simulink model "Model_6DoF_Complete"  (R2024a)
settings: Solver=VariableStepAuto  StartTime=0.0  StopTime=6  RelTol=1e-5
model workspace: external: MATLAB File C:\Users\C27Derek.Weissinger\OneDrive - USAFA (AFAcademy.AF.edu)\Documents\Classes\Summer 26\Astro 499\Derek-Weissinger-GNC-Methods-2026\MATLAB + Simulink\vehicle_params.m (data not in the file)
undefined symbols (not defined in the file): I, Kd, Ki, Kp, Lg, m, psii, thetai, Ts
libraries: simulink_extras x10, eeGeneralControl x2, sharedtransform x2, shared6dof x1, sharedutil x1
settings Model: Creator=C28Derek.Weissinger  LastModifiedBy=C28Derek.Weissinger

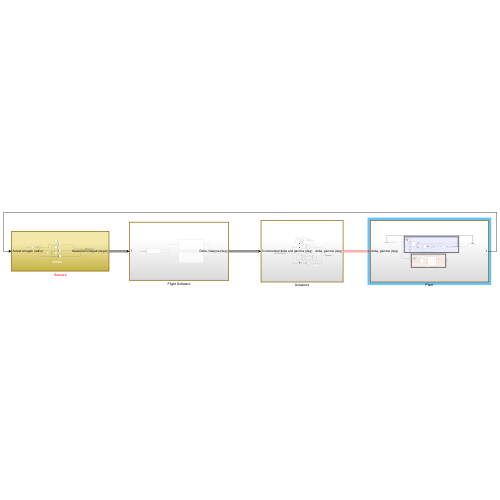
[thumbnail: Simulink's stored preview of the top-level diagram]
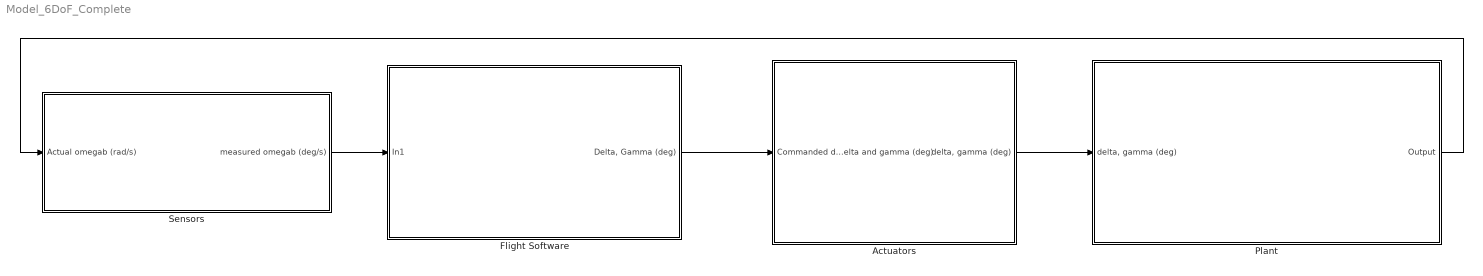
== system Model_6DoF_Complete ==
  Actuators : Subsystem
  Flight Software : Subsystem
  Plant : Subsystem
  Sensors : Subsystem
  wires:
  Plant/1(Output) -> Sensors/1(Actual omegab (rad/s))
  Sensors/1(measured omegab (deg/s)) -> Flight Software/1(In1)
  Flight Software/1("Delta, Gamma (deg)") -> Actuators/1(Commanded delta and gamma (deg))
  Actuators/1("delta, gamma (deg)") -> Plant/1("delta, gamma (deg)")

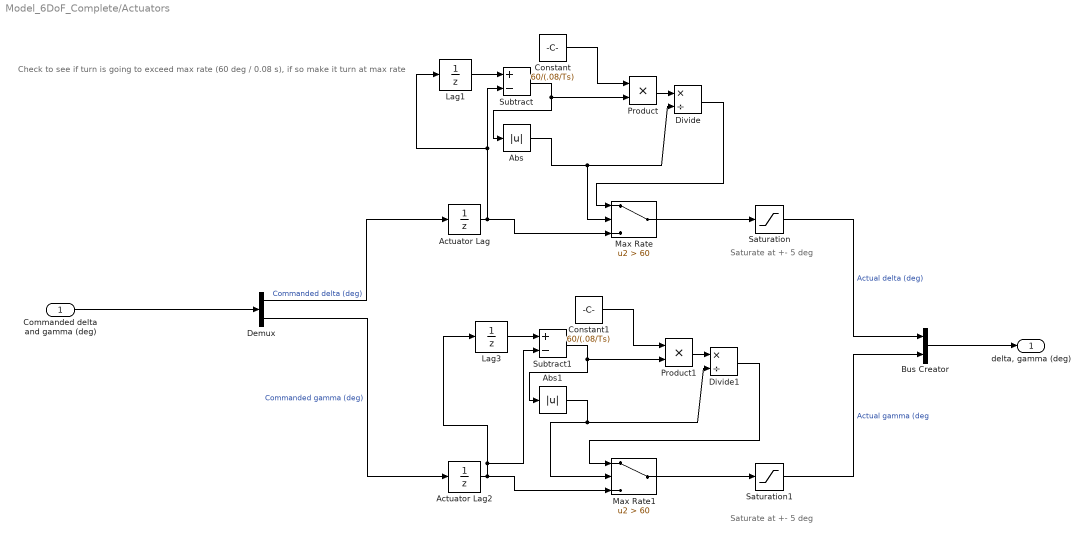
== system Model_6DoF_Complete/Actuators ==
  note: Saturate at +- 5 deg
  note: Check to see if turn is going to exceed max rate (60 deg / 0.08 s), if so make it turn at max rate
  note: Saturate at +- 5 deg
  Commanded delta and gamma (deg) : Inport
  Abs : Abs  SaturateOnIntegerOverflow=off
  Abs1 : Abs  SaturateOnIntegerOverflow=off
  Actuator Lag : UnitDelay  SampleTime=Ts  HasFrameUpgradeWarning=on
  Actuator Lag2 : UnitDelay  SampleTime=Ts  HasFrameUpgradeWarning=on
  Bus Creator : BusCreator  Inputs=2
  Constant : Constant  Value=60/(.08/Ts)
  Constant1 : Constant  Value=60/(.08/Ts)
  Demux : Demux  Outputs=2
  Divide : Product  Inputs=*/
  Divide1 : Product  Inputs=*/
  Lag1 : UnitDelay  SampleTime=0.08  HasFrameUpgradeWarning=on
  Lag3 : UnitDelay  SampleTime=0.08  HasFrameUpgradeWarning=on
  Max Rate : Switch  Criteria=u2 > Threshold  Threshold=60  SaturateOnIntegerOverflow=off  InputSameDT=off
  Max Rate1 : Switch  Criteria=u2 > Threshold  Threshold=60  SaturateOnIntegerOverflow=off  InputSameDT=off
  Product : Product
  Product1 : Product
  Saturation : Saturate  UpperLimit=5  LowerLimit=-5
  Saturation1 : Saturate  UpperLimit=5  LowerLimit=-5
  Subtract : Sum  Inputs=+-
  Subtract1 : Sum  Inputs=+-
  "delta, gamma (deg)" : Outport
  wires:
  Actuator Lag/1 -> Max Rate/3, Subtract/2, Lag1/1
  Lag1/1 -> Subtract/1
  Subtract/1 -> Abs/1, Product/2
  Abs/1 -> Max Rate/2, Divide/2
  Constant/1 -> Product/1
  Product/1 -> Divide/1
  Max Rate/1 -> Saturation/1
  Saturation1/1 -> Bus Creator/2  "Actual gamma (deg"
  Max Rate1/1 -> Saturation1/1
  Subtract1/1 -> Abs1/1, Product1/2
  Abs1/1 -> Max Rate1/2, Divide1/2
  Actuator Lag2/1 -> Max Rate1/3, Subtract1/2, Lag3/1
  Demux/2 -> Actuator Lag2/1  "Commanded gamma (deg)"
  Product1/1 -> Divide1/1
  Constant1/1 -> Product1/1
  Lag3/1 -> Subtract1/1
  Demux/1 -> Actuator Lag/1  "Commanded delta (deg)"
  Commanded delta and gamma (deg)/1 -> Demux/1
  Bus Creator/1 -> "delta, gamma (deg)"/1
  Saturation/1 -> Bus Creator/1  "Actual delta (deg)"
  Divide1/1 -> Max Rate1/1
  Divide/1 -> Max Rate/1

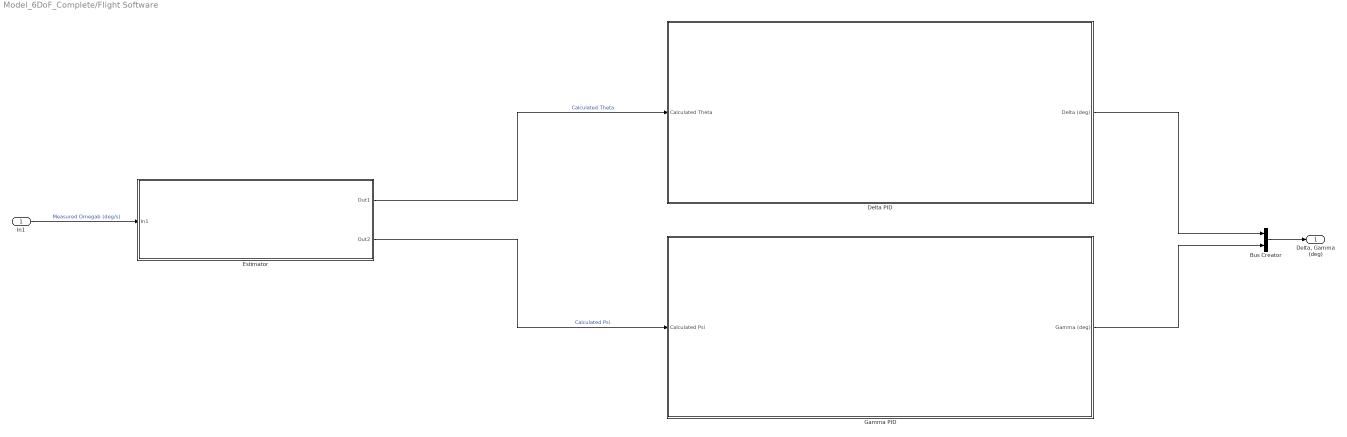
== system Model_6DoF_Complete/Flight Software ==
  In1 : Inport
  Bus Creator : BusCreator  Inputs=2
  Delta PID : Subsystem
  Estimator : Subsystem
  Gamma PID : Subsystem
  "Delta, Gamma (deg)" : Outport
  wires:
  In1/1 -> Estimator/1(In1)  "Measured Omegab (deg/s)"
  Bus Creator/1 -> "Delta, Gamma (deg)"/1
  Delta PID/1(Delta (deg)) -> Bus Creator/1
  Gamma PID/1(Gamma (deg)) -> Bus Creator/2
  Estimator/1(Out1) -> Delta PID/1(Calculated Theta)  "Calculated Theta"
  Estimator/2(Out2) -> Gamma PID/1(Calculated Psi)  "Calculated Psi"

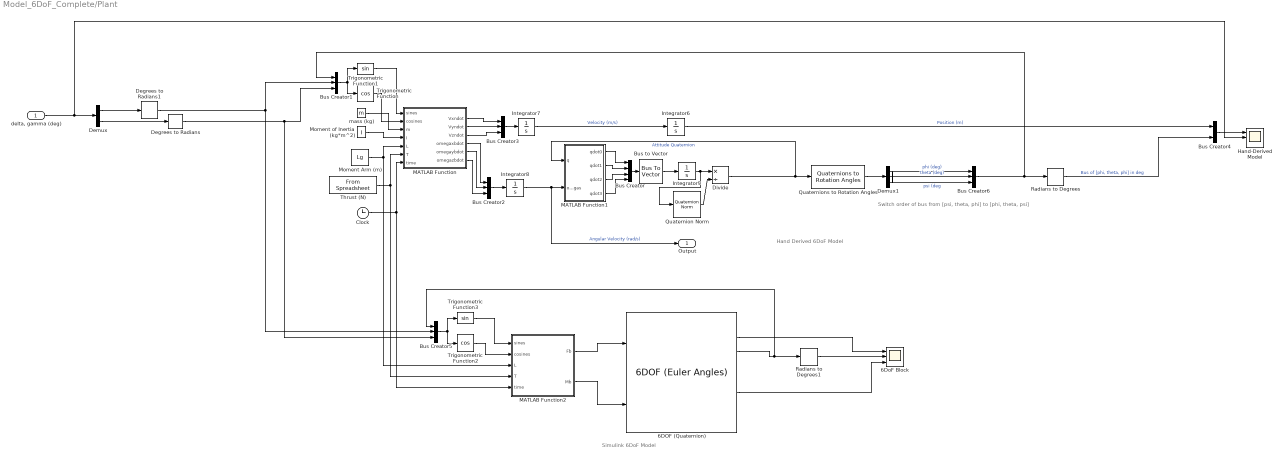
== system Model_6DoF_Complete/Plant ==
  note: Hand Derived 6DoF Model
  note: Simulink 6DoF Model
  note: Switch order of bus from [psi, theta, phi] to [phi, theta, psi]
  "delta, gamma (deg)" : Inport
  6DOF (Quaternion) : shared6dof/6DOF (Euler Angles)  units=Metric (MKS)  mtype=Fixed  rep=Quaternion  xme_0=[0 0 0]  Vm_0=[0 0 0]  eul_0=[0 deg2rad(thetai) deg2rad(psii)]  pm_0=[0 0 0]  mass_0=m  mass_e=0.5  mass_f=2.0  inertia=eye(3) * I  inertia_e=eye(3)  inertia_f=2*eye(3)  k_quat=1.0  vre_flag=on  abi_flag=off  aMode=0  xme_statename=''  Vm_statename=''  eul_statename=''  quat_statename=''  pm_statename=''  mass_statename=''
      settings: LibrarySourceBlock=aerolib6dof2/6DOF (Quaternion)
  6DoF Block : Scope  NumInputPorts=3
  Bus Creator : BusCreator  Inputs=4
  Bus Creator{1..3,5..6} (5 alike) : BusCreator  Inputs=3
  Bus Creator4 : BusCreator  Inputs=2
  Bus to Vector : BusToVector
  Clock : Clock
  Degrees to Radians : simulink_extras/Transformations/Degrees to Radians
  Degrees to Radians1 : simulink_extras/Transformations/Degrees to Radians
  Demux : Demux  Outputs=2
  Demux1 : Demux  Outputs=3
  Divide : Product  Inputs=*/
  Hand-Derived Model : Scope  NumInputPorts=3
  Integrator6 : Integrator
  Integrator7 : Integrator  InitialCondition=[0, 0, 0]
  Integrator8 : Integrator  InitialCondition=[0, 0, 0]
  Integrator9 : Integrator  InitialCondition=eul2quat([deg2rad(psii),deg2rad(thetai),deg2rad(0)])
  MATLAB Function : MATLAB Function  TreatAsAtomicUnit=on
  MATLAB Function1 : MATLAB Function  TreatAsAtomicUnit=on
  MATLAB Function2 : MATLAB Function  TreatAsAtomicUnit=on
  Moment Arm (m) : Constant  Value=Lg
  Moment of Inertia (kg*m^2) : Constant  Value=I
  Quaternion Norm : sharedutil/Quaternion Norm  aMode=aMode
      settings: LibrarySourceBlock=|
      | aerolibutil/Quaternion
      | Norm
  Quaternions to Rotation Angles : sharedtransform/Quaternions to Rotation Angles  rotationOrder=ZYX  aMode=aMode
  Radians to Degrees : simulink_extras/Transformations/Radians to Degrees
  Radians to Degrees1 : simulink_extras/Transformations/Radians to Degrees
  Thrust (N) : FromSpreadsheet  FileName=Estes_F15.csv  SheetName=Estes_F15  ExtrapolationAfterLastDataPoint=Ground value
  Trigonometric Function : Trigonometry  Operator=cos
  Trigonometric Function1 : Trigonometry
  Trigonometric Function2 : Trigonometry  Operator=cos
  Trigonometric Function3 : Trigonometry
  mass (kg) : Constant  Value=m
  Output : Outport
  wires:
  "delta, gamma (deg)"/1 -> Hand-Derived Model/2, Demux/1
  Moment Arm (m)/1 -> MATLAB Function2/3(L), MATLAB Function/5(L)
  Moment of Inertia (kg*m^2)/1 -> MATLAB Function/4(I)
  Degrees to Radians/1 -> Bus Creator5/3, Bus Creator1/3
  Bus Creator1/1 -> Trigonometric Function/1, Trigonometric Function1/1
  Trigonometric Function1/1 -> MATLAB Function/1(sines)
  Trigonometric Function/1 -> MATLAB Function/2(cosines)
  Thrust (N)/1 -> MATLAB Function2/4(T), MATLAB Function/6(T)
  mass (kg)/1 -> MATLAB Function/3(m)
  MATLAB Function/1(Vxndot) -> Bus Creator3/1
  Integrator7/1 -> Integrator6/1  "Velocity (m/s)"
  Integrator6/1 -> Bus Creator4/1  "Position (m)"
  Integrator8/1 -> Output/1, MATLAB Function1/2(omegas)  "Angular Velocity (rad/s)"
  MATLAB Function1/1(qdot0) -> Bus Creator/1
  Bus Creator4/1 -> Hand-Derived Model/1
  Clock/1 -> MATLAB Function2/5(time), MATLAB Function/7(time)
  Degrees to Radians1/1 -> Bus Creator1/2, Bus Creator5/2
  MATLAB Function1/2(qdot1) -> Bus Creator/2
  MATLAB Function1/3(qdot2) -> Bus Creator/3
  MATLAB Function1/4(qdot3) -> Bus Creator/4
  Bus Creator/1 -> Bus to Vector/1
  Bus to Vector/1 -> Integrator9/1
  Bus Creator2/1 -> Integrator8/1
  MATLAB Function/4(omegaxbdot) -> Bus Creator2/1
  MATLAB Function/5(omegaybdot) -> Bus Creator2/2
  MATLAB Function/6(omegazbdot) -> Bus Creator2/3
  Bus Creator3/1 -> Integrator7/1
  MATLAB Function/2(Vyndot) -> Bus Creator3/2
  MATLAB Function/3(Vzndot) -> Bus Creator3/3
  Integrator9/1 -> Quaternion Norm/1, Divide/1
  Divide/1 -> MATLAB Function1/1(q), Quaternions to Rotation Angles/1  "Attitude Quaternion"
  Quaternion Norm/1 -> Divide/2
  Demux/2 -> Degrees to Radians/1
  Demux/1 -> Degrees to Radians1/1
  MATLAB Function2/1(Fb) -> 6DOF (Quaternion)/1
  MATLAB Function2/2(Mb) -> 6DOF (Quaternion)/2
  6DOF (Quaternion)/3 -> Bus Creator5/1, Radians to Degrees1/1
  Radians to Degrees1/1 -> 6DoF Block/2
  6DOF (Quaternion)/2 -> 6DoF Block/1
  6DOF (Quaternion)/6 -> 6DoF Block/3
  Bus Creator5/1 -> Trigonometric Function2/1, Trigonometric Function3/1
  Trigonometric Function3/1 -> MATLAB Function2/1(sines)
  Trigonometric Function2/1 -> MATLAB Function2/2(cosines)
  Radians to Degrees/1 -> Bus Creator4/2  "Bus of [phi, theta, phi] in deg"
  Demux1/2 -> Bus Creator6/2  "theta (deg)"
  Demux1/3 -> Bus Creator6/1  "phi (deg)"
  Demux1/1 -> Bus Creator6/3  "psi (deg"
  Quaternions to Rotation Angles/1 -> Demux1/1
  Bus Creator6/1 -> Bus Creator1/1, Radians to Degrees/1

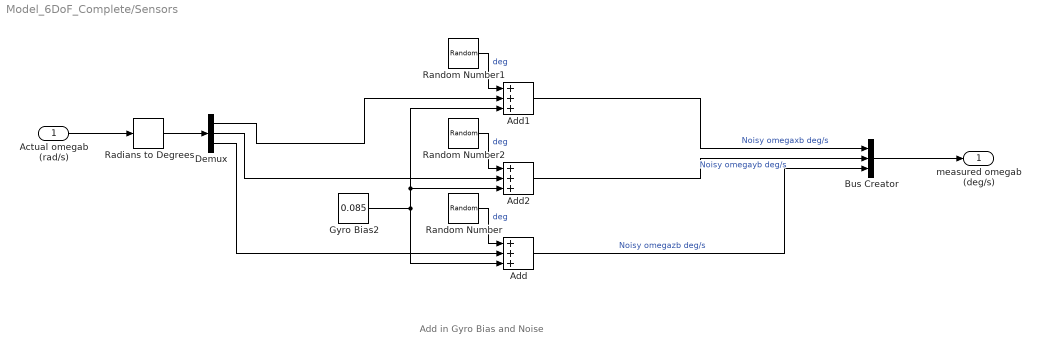
== system Model_6DoF_Complete/Sensors ==
  note: Add in Gyro Bias and Noise
  Actual omegab (rad/s) : Inport
  Add : Sum  Inputs=+++
  Add1 : Sum  Inputs=+++
  Add2 : Sum  Inputs=+++
  Bus Creator : BusCreator  Inputs=3
  Demux : Demux  Outputs=3
  Gyro Bias2 : Constant  Value=0.085
  Radians to Degrees : simulink_extras/Transformations/Radians to Degrees
  Random Number : RandomNumber  Seed=3  SampleTime=0.01
  Random Number1 : RandomNumber  Seed=1  SampleTime=0.01
  Random Number2 : RandomNumber  Seed=2  SampleTime=0.01
  measured omegab (deg/s) : Outport
  wires:
  Actual omegab (rad/s)/1 -> Radians to Degrees/1
  Random Number/1 -> Add/1  "deg"
  Add/1 -> Bus Creator/3  "Noisy omegazb deg/s"
  Bus Creator/1 -> measured omegab (deg/s)/1
  Add1/1 -> Bus Creator/1  "Noisy omegaxb deg/s"
  Random Number1/1 -> Add1/1  "deg"
  Gyro Bias2/1 -> Add1/3, Add2/3, Add/3
  Add2/1 -> Bus Creator/2  "Noisy omegayb deg/s"
  Random Number2/1 -> Add2/1  "deg"
  Demux/1 -> Add1/2
  Demux/2 -> Add2/2
  Demux/3 -> Add/2
  Radians to Degrees/1 -> Demux/1

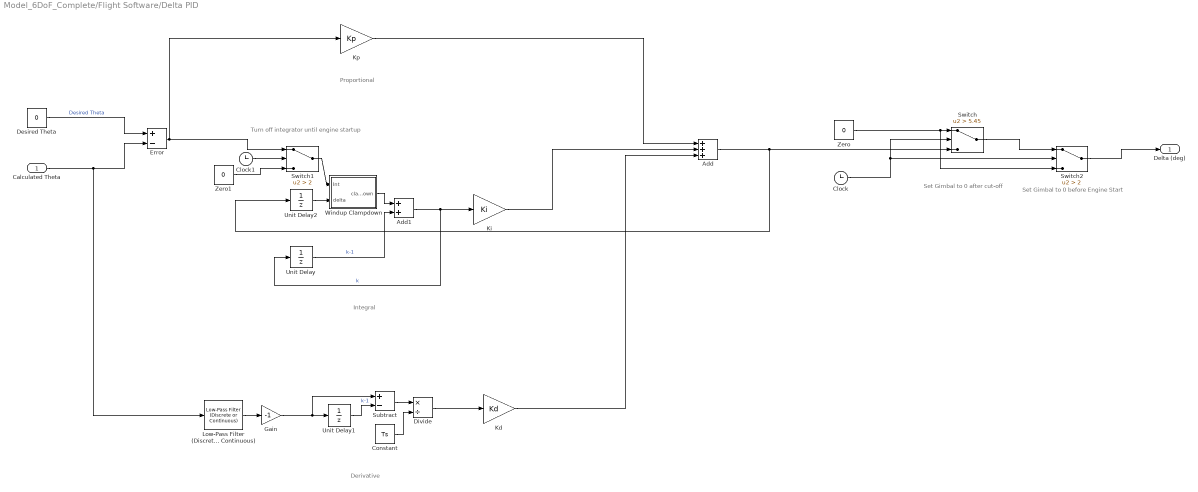
== system Model_6DoF_Complete/Flight Software/Delta PID ==
  note: Turn off integrator until engine startup
  note: Integral
  note: Proportional
  note: Derivative
  note: Set Gimbal to 0 before Engine Start
  note: Set Gimbal to 0 after cut-off
  Calculated Theta : Inport
  Add : Sum  Inputs=+++
  Add1 : Sum
  Clock : Clock
  Clock1 : Clock
  Constant : Constant  Value=Ts
  Desired Theta : Constant  Value=0
  Divide : Product  Inputs=*/
  Error : Sum  Inputs=+-
  Gain : Gain  Gain=-1
  Kd : Gain  Gain=Kd
  Ki : Gain  Gain=Ki
  Kp : Gain  Gain=Kp
  Low-Pass Filter (Discrete or Continuous) : eeGeneralControl/Low-Pass Filter (Discrete or Continuous)  K=1  T=2*Ts  B=inf  A=-inf  init_option=Inherited from block input  x0=0  Ts=-1
  Subtract : Sum  Inputs=+-
  Switch : Switch  Criteria=u2 > Threshold  Threshold=5.45  SaturateOnIntegerOverflow=off  InputSameDT=off
  Switch1 : Switch  Criteria=u2 > Threshold  Threshold=2  SaturateOnIntegerOverflow=off  InputSameDT=off
  Switch2 : Switch  Criteria=u2 > Threshold  Threshold=2  SaturateOnIntegerOverflow=off  InputSameDT=off
  Unit Delay : UnitDelay  SampleTime=Ts  HasFrameUpgradeWarning=on
  Unit Delay1 : UnitDelay  SampleTime=Ts  HasFrameUpgradeWarning=on
  Unit Delay2 : UnitDelay  SampleTime=Ts  HasFrameUpgradeWarning=on
  Windup Clampdown : MATLAB Function  TreatAsAtomicUnit=on
  Zero : Constant  Value=0  OutDataTypeStr=Inherit: Inherit via back propagation
  Zero1 : Constant  Value=0  OutDataTypeStr=Inherit: Inherit via back propagation
  Delta (deg) : Outport
  wires:
  Desired Theta/1 -> Error/1  "Desired Theta"
  Subtract/1 -> Divide/1
  Add1/1 -> Unit Delay/1, Ki/1  "k"
  Unit Delay1/1 -> Subtract/2  "k-1"
  Error/1 -> Switch1/1, Kp/1
  Switch/1 -> Switch2/1
  Unit Delay/1 -> Add1/2  "k-1"
  Divide/1 -> Kd/1
  Zero/1 -> Switch2/3, Switch/1
  Kd/1 -> Add/3
  Kp/1 -> Add/1
  Gain/1 -> Subtract/1, Unit Delay1/1
  Clock/1 -> Switch2/2, Switch/2
  Switch2/1 -> Delta (deg)/1
  Constant/1 -> Divide/2
  Calculated Theta/1 -> Low-Pass Filter (Discrete or Continuous)/1, Error/2
  Ki/1 -> Add/2
  Switch1/1 -> Windup Clampdown/1(Int)
  Clock1/1 -> Switch1/2
  Zero1/1 -> Switch1/3
  Add/1 -> Unit Delay2/1, Switch/3
  Windup Clampdown/1(clampdown) -> Add1/1
  Low-Pass Filter (Discrete or Continuous)/1 -> Gain/1
  Unit Delay2/1 -> Windup Clampdown/2(delta)

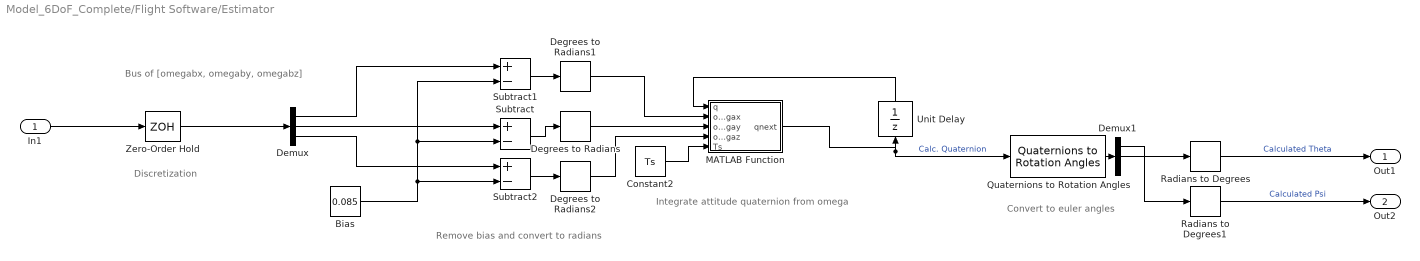
== system Model_6DoF_Complete/Flight Software/Estimator ==
  note: Bus of [omegabx, omegaby, omegabz]
  note: Convert to euler angles
  note: Discretization
  note: Remove bias and convert to radians
  note: Integrate attitude quaternion from omega
  In1 : Inport
  Bias : Constant  Value=0.085  SampleTime=Ts
  Constant2 : Constant  Value=Ts
  Degrees to Radians : simulink_extras/Transformations/Degrees to Radians
  Degrees to Radians1 : simulink_extras/Transformations/Degrees to Radians
  Degrees to Radians2 : simulink_extras/Transformations/Degrees to Radians
  Demux : Demux  Outputs=3
  Demux1 : Demux  Outputs=3
  MATLAB Function : MATLAB Function  TreatAsAtomicUnit=on
  Quaternions to Rotation Angles : sharedtransform/Quaternions to Rotation Angles  rotationOrder=ZYX  aMode=aMode
  Radians to Degrees : simulink_extras/Transformations/Radians to Degrees
  Radians to Degrees1 : simulink_extras/Transformations/Radians to Degrees
  Subtract : Sum  Inputs=+-
  Subtract1 : Sum  Inputs=+-
  Subtract2 : Sum  Inputs=+-
  Unit Delay : UnitDelay  InitialCondition=eul2quat([deg2rad(psii),deg2rad(thetai),0])  SampleTime=Ts  HasFrameUpgradeWarning=on
  Zero-Order Hold : ZeroOrderHold  SampleTime=Ts
  Out1 : Outport
  Out2 : Outport  Port=2
  wires:
  Degrees to Radians/1 -> MATLAB Function/3(omegay)
  In1/1 -> Zero-Order Hold/1
  Constant2/1 -> MATLAB Function/5(Ts)
  Quaternions to Rotation Angles/1 -> Demux1/1
  MATLAB Function/1(qnext) -> Quaternions to Rotation Angles/1, Unit Delay/1  "Calc. Quaternion"
  Unit Delay/1 -> MATLAB Function/1(q)
  Zero-Order Hold/1 -> Demux/1
  Demux1/2 -> Radians to Degrees/1
  Bias/1 -> Subtract2/2, Subtract1/2, Subtract/2
  Subtract/1 -> Degrees to Radians/1
  Demux/1 -> Subtract1/1
  Demux/2 -> Subtract/1
  Demux/3 -> Subtract2/1
  Subtract1/1 -> Degrees to Radians1/1
  Subtract2/1 -> Degrees to Radians2/1
  Degrees to Radians2/1 -> MATLAB Function/4(omegaz)
  Degrees to Radians1/1 -> MATLAB Function/2(omegax)
  Demux1/1 -> Radians to Degrees1/1
  Radians to Degrees/1 -> Out1/1  "Calculated Theta"
  Radians to Degrees1/1 -> Out2/1  "Calculated Psi"

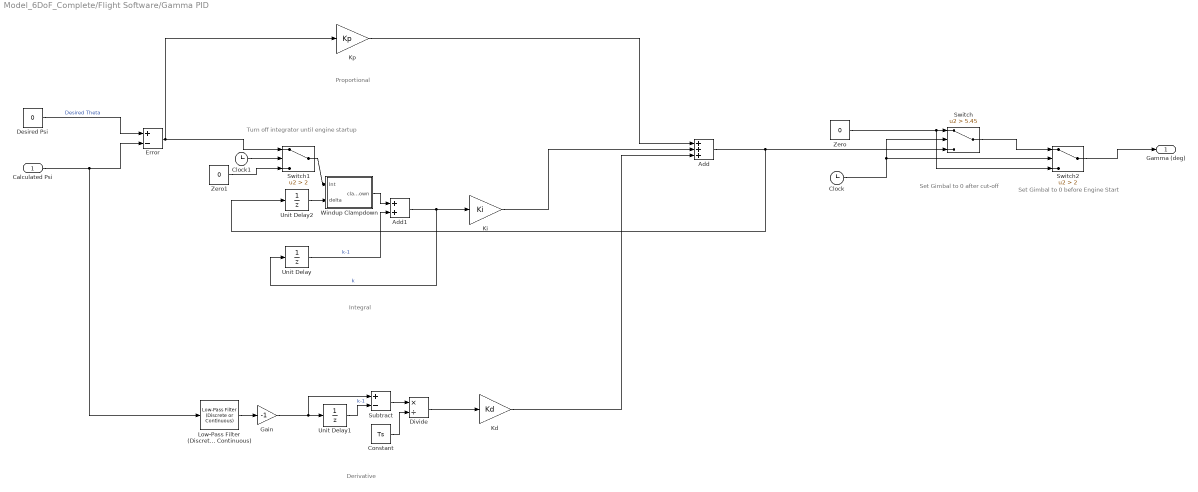
== system Model_6DoF_Complete/Flight Software/Gamma PID ==
  note: Turn off integrator until engine startup
  note: Integral
  note: Proportional
  note: Derivative
  note: Set Gimbal to 0 before Engine Start
  note: Set Gimbal to 0 after cut-off
  Calculated Psi : Inport
  Add : Sum  Inputs=+++
  Add1 : Sum
  Clock : Clock
  Clock1 : Clock
  Constant : Constant  Value=Ts
  Desired Psi : Constant  Value=0
  Divide : Product  Inputs=*/
  Error : Sum  Inputs=+-
  Gain : Gain  Gain=-1
  Kd : Gain  Gain=Kd
  Ki : Gain  Gain=Ki
  Kp : Gain  Gain=Kp
  Low-Pass Filter (Discrete or Continuous) : eeGeneralControl/Low-Pass Filter (Discrete or Continuous)  K=1  T=2*Ts  B=inf  A=-inf  init_option=Inherited from block input  x0=0  Ts=-1
  Subtract : Sum  Inputs=+-
  Switch : Switch  Criteria=u2 > Threshold  Threshold=5.45  SaturateOnIntegerOverflow=off  InputSameDT=off
  Switch1 : Switch  Criteria=u2 > Threshold  Threshold=2  SaturateOnIntegerOverflow=off  InputSameDT=off
  Switch2 : Switch  Criteria=u2 > Threshold  Threshold=2  SaturateOnIntegerOverflow=off  InputSameDT=off
  Unit Delay : UnitDelay  SampleTime=Ts  HasFrameUpgradeWarning=on
  Unit Delay1 : UnitDelay  SampleTime=Ts  HasFrameUpgradeWarning=on
  Unit Delay2 : UnitDelay  SampleTime=Ts  HasFrameUpgradeWarning=on
  Windup Clampdown : MATLAB Function  TreatAsAtomicUnit=on
  Zero : Constant  Value=0  OutDataTypeStr=Inherit: Inherit via back propagation
  Zero1 : Constant  Value=0  OutDataTypeStr=Inherit: Inherit via back propagation
  Gamma (deg) : Outport
  wires:
  Desired Psi/1 -> Error/1  "Desired Theta"
  Subtract/1 -> Divide/1
  Add1/1 -> Unit Delay/1, Ki/1  "k"
  Unit Delay1/1 -> Subtract/2  "k-1"
  Error/1 -> Switch1/1, Kp/1
  Switch/1 -> Switch2/1
  Unit Delay/1 -> Add1/2  "k-1"
  Divide/1 -> Kd/1
  Zero/1 -> Switch2/3, Switch/1
  Kd/1 -> Add/3
  Kp/1 -> Add/1
  Gain/1 -> Subtract/1, Unit Delay1/1
  Clock/1 -> Switch2/2, Switch/2
  Switch2/1 -> Gamma (deg)/1
  Constant/1 -> Divide/2
  Calculated Psi/1 -> Low-Pass Filter (Discrete or Continuous)/1, Error/2
  Ki/1 -> Add/2
  Switch1/1 -> Windup Clampdown/1(Int)
  Clock1/1 -> Switch1/2
  Zero1/1 -> Switch1/3
  Add/1 -> Unit Delay2/1, Switch/3
  Windup Clampdown/1(clampdown) -> Add1/1
  Low-Pass Filter (Discrete or Continuous)/1 -> Gain/1
  Unit Delay2/1 -> Windup Clampdown/2(delta)

== matlab function Model_6DoF_Complete/Flight Software/Gamma PID/Windup Clampdown ==
  data: Int input; clampdown output; delta input
function clampdown = fcn(Int,delta)
%Signs are different than what you would usually expect because of how we
%defined + rotation about y axis.
if abs(Int) > 5 && Int*delta > 0 
        clampdown = 0;
else
    clampdown = Int;
end
end

== matlab function Model_6DoF_Complete/Plant/MATLAB Function2 ==
  data: sines input; Fb output double size=3; cosines input; L input; T input size=1; Mb output size=3; time input
function [Fb, Mb] = F_and_M_Block(sines, cosines, L, T, time)
% Inputs:
% sines: 5x1 vector of the sine of phi, sine of theta, sine of psi, sine of
% delta, and sine of gamma, in that order.
% cosines: 5x1 vector of the cosine of phi, cosine of theta, cosine of psi, 
% cosine of delta, and cosine of gamma,  in that order.
% delta: Gimbal Angle wrt pitch (rad)
% gamma: Gimbal Angle wrt yaw (rad)
% L: Length from rocket's CG to point of thrust (m).
% T: scalar magnitude of thrust (N)
% time: model time (s)
% Outputs:
% Vndot: 3x1 vector of linear acceleration wrt. the navigation frame.
% omegandot: 3x1 vector of angular acceleration wrt. the navigation frame.

g = 9.81; %gravitational constant, m/s^2.

%define shorthand variables to make typing easier
sph = sines(1);
sth = sines(2);
sps = sines(3);
sde = sines(4);
sga = sines(5);
cph = cosines(1);
cth = cosines(2);
cps = cosines(3);
cde = cosines(4);
cga = cosines(5);

% Coordinate Frames: body frame (b) of rocket (x is dir. of nose, y is pitch
% axis., z is yaw axis. right-handed) to nav. frame (n) (+x is up, +y is east, 
% +z is north) via a passive 321 rotation.
%6DoF Nav. Frame (e): x+ is north, y+ is east, z+ is down
%Therefore, our desired DCM from n frame to e frame is a 90 deg clockwise
%rotation abt. the y axis

R_en = [[0; 0; 1], [0; 1; 0], [-1; 0; 0]];

R_nb = [cps*cth, -cth*sps, sth; 
        -cps*sph*sth+cph*sps, cth*cps+sph*sps*sth, cth*sph;
        -sph*sps-cph*cps*sth, cph*sps*sth-cps*sph, cph*cth]; 

R_eb = R_en * R_nb;

%3x1 vector representing the thrust vector in the body frame
Tb = T * [cde*cga; sga; -sde]; 
%3x1 vector finding sum of forces in body frame, N
%If statement simulates engine startup at time = 2s
if time > 2
    Fb = R_en' * (Tb + (R_nb' * [-g; 0; 0]));
else
    Fb = R_en' * Tb;
end

%3x1 vector encoding torque in the body frame, N*m
Mb = (T*L) * [0; sde; sga];

end

== matlab function Model_6DoF_Complete/Flight Software/Delta PID/Windup Clampdown ==
  data: Int input; clampdown output; delta input
function clampdown = fcn(Int,delta)
%Signs are different than what you would usually expect because of how we
%defined + rotation about y axis.
if abs(Int) > 5 && Int*delta > 0 
        clampdown = 0;
else
    clampdown = Int;
end
end

== matlab function Model_6DoF_Complete/Plant/MATLAB Function ==
  data: sines input; Vxndot output double size=1; cosines input; m input; I input; L input; T input size=1; Vyndot output size=1; time input; Vzndot output size=1; omegaxbdot output size=1; omegaybdot output size=1; omegazbdot output size=1
function [Vxndot, Vyndot, Vzndot, omegaxbdot, omegaybdot, omegazbdot] = EoM(sines, cosines, m, I, L, T, time)
% Inputs:
% sines: 5x1 vector of the sine of phi, sine of theta, sine of psi, sine of
% delta, and sine of gamma, in that order.
% cosines: 5x1 vector of the cosine of phi, cosine of theta, cosine of psi, 
% cosine of delta, and cosine of gamma,  in that order.
% delta: Gimbal Angle wrt pitch (rad)
% gamma: Gimbal Angle wrt yaw (rad)
% m: mass of rocket (kg)
% I: moment of inertia wrt to pitch and yaw (kg*m^2). For our model, 
% we assume I_yy = I_zz
% L: Length from rocket's CG to point of thrust (m).
% T: scalar magnitude of thrust (N)
% time: model time (s)
% Outputs:
% Vndot: 3x1 vector of linear acceleration wrt. the navigation frame.
% omegandot: 3x1 vector of angular acceleration wrt. the navigation frame.
Vndot = zeros(3,1);
omegandot = zeros(3,1);

g = 9.81; %gravitational constant, m/s^2.

%define shorthand variables to make typing easier
sph = sines(1);
sth = sines(2);
sps = sines(3);
sde = sines(4);
sga = sines(5);
cph = cosines(1);
cth = cosines(2);
cps = cosines(3);
cde = cosines(4);
cga = cosines(5);

%DCM converting from body frame of rocket (x is dir. of nose, y is pitch
% dir., z is yaw dir. right-handed) to nav. frame (+x is up, +y is east, 
% +z is north) via a passive 321 rotation.
R_nb = [cps*cth, -cth*sps, sth; 
        -cps*sph*sth+cph*sps, cth*cps+sph*sps*sth, cth*sph;
        -sph*sps-cph*cps*sth, cph*sps*sth-cps*sph, cph*cth]; 

%3x1 vector representing the thrust vector in the body frame
Tb = T * [cde*cga; sga; -sde]; 

Tn = R_nb * Tb / m; %Convert to nav. frame

% if time > 2 %Disable gravity before engine comes online, simulate sitting at the pad
%     Vndot = Tn/m - [g;0;0];
% else
%     Vndot = Tn/m;
% end

Vndot = Tn/m;
%Check if the rocket is still on the pad, engine startup at t=2 sec
if time > 2
Vxndot = Vndot(1) - g;
else
Vxndot = Vndot(1);
end

Vyndot = Vndot(2);
Vzndot = Vndot(3);

%3x1 vector encoding angular acceleration in body frame, rad/s
omegabdot = (T*L/I) * [0; sde; sga];
omegaxbdot = omegabdot(1);
omegaybdot = omegabdot(2);
omegazbdot = omegabdot(3);
end

== matlab function Model_6DoF_Complete/Plant/MATLAB Function1 ==
  data: q input; omegas input; qdot0 output; qdot1 output; qdot2 output; qdot3 output
function [qdot0, qdot1, qdot2, qdot3] = QuatDeriv(q, omegas)
% Input:
% q: Current attitude quaternion (real part first)
% Omegas: 3x1 vector of omegaxn, omegayn, omegazn, in that order
% Output: qdot: derivative of attitude, expressed as quaternion, will be
% subsequently integrated to get new attitude.

omegaxn = omegas(1);
omegayn = omegas(2);
omegazn = omegas(3);

omegamatrix = [0 -omegaxn -omegayn -omegazn;
               omegaxn 0 omegazn -omegayn;
               omegayn -omegazn 0 omegaxn;
               omegazn omegayn -omegaxn 0];

% qmatrix = [q0 -q3 q2 q1;
%           q3 q0 -q1 q2;
%           -q2 q1 q0 q3;
%           -q1 -q2 -q3 q0];
% omega = [omegax; omegay; omegaz; 0];
% qdot = 0.5 * matrix * omega;

qdot = 0.5 * omegamatrix * q;
qdot0 = qdot(1);
qdot1 = qdot(2);
qdot2 = qdot(3);
qdot3 = qdot(4);

== matlab function Model_6DoF_Complete/Flight Software/Estimator/MATLAB Function ==
  data: q input size=4; omegax input; omegay input; omegaz input; qnext output size=4; Ts input
function qnext = fcn(q, omegax, omegay, omegaz, Ts)
%Closed form of quaternion integrator, as found on 
% https://ahrs.readthedocs.io/en/latest/filters/angular.html

omegamatrix = [0 -omegax -omegay -omegaz;
               omegax 0 omegaz -omegay;
               omegay -omegaz 0 omegax;
               omegaz omegay -omegax 0];

qdot = 0.5 * omegamatrix * q;
qnext = q + qdot*Ts;
qnext = qnext/norm(qnext);

end
